simulink model "example1_0511"  (R2023b)
settings: Solver=VariableStepAuto  StartTime=0.0  StopTime=10.0  RelTol=1e-3
settings Model: Creator=martinhaugen  LastModifiedBy=martinhaugen

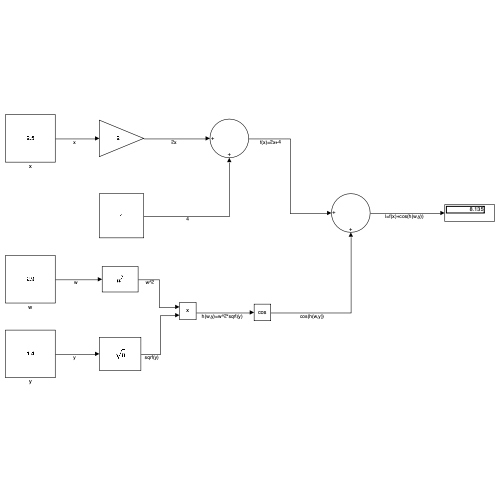
[thumbnail: Simulink's stored preview of the top-level diagram]
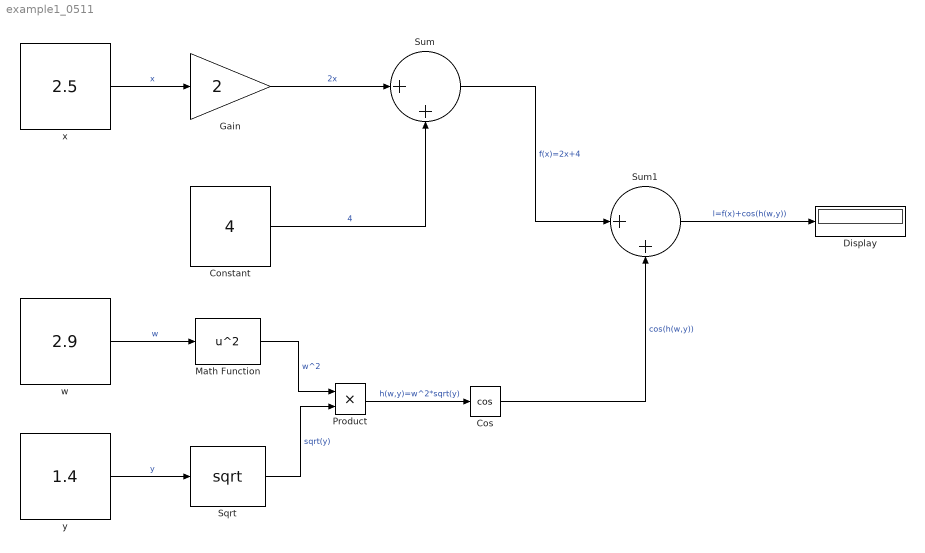
== system example1_0511 ==
  Constant : Constant  Value=4
  Cos : Trigonometry  Operator=cos
  Display : Display
  Gain : Gain  Gain=2
  Math Function : Math  Operator=square
  Product : Product
  Sqrt : Sqrt
  Sum : Sum  Inputs=|++
  Sum1 : Sum  Inputs=|++
  w : Constant  Value=2.9
  x : Constant  Value=2.5
  y : Constant  Value=1.4
  wires:
  x/1 -> Gain/1  "x"
  Gain/1 -> Sum/1  "2x"
  Constant/1 -> Sum/2  "4"
  w/1 -> Math Function/1  "w"
  y/1 -> Sqrt/1  "y"
  Math Function/1 -> Product/1  "w^2"
  Sqrt/1 -> Product/2  "sqrt(y)"
  Product/1 -> Cos/1  "h(w,y)=w^2*sqrt(y)"
  Cos/1 -> Sum1/2  "cos(h(w,y))"
  Sum/1 -> Sum1/1  "f(x)=2x+4"
  Sum1/1 -> Display/1  "l=f(x)+cos(h(w,y))"
